simulink model "simulink_model"  (R2015a)
settings: Solver=ode45  StartTime=0.0  StopTime=20  RelTol=1e-3
values from neighbouring files (symbols this model uses):
  g = 9.8    [init_tp.m]    (also in init_tp3.m)
  J = 0.02    [init_tp.m]    (also in init_tp3.m)
  K = place(A,B,p)    [init_tp.m]    (also in init_tp3.m)
  K2 = place(A2,B2,p2)    [init_tp.m]    (also in init_tp3.m)
  m = 0.6    [init_tp.m]    (also in init_tp3.m)
  sigma = 0.8    [init_tp.m]    (also in init_tp3.m)
  w = ((m*g*g)/((1+sigma)*J))^(1/4)    (= 6.32521402527)    [init_tp.m]    (also in init_tp3.m)
settings Model: Creator=root  LastModifiedBy=root

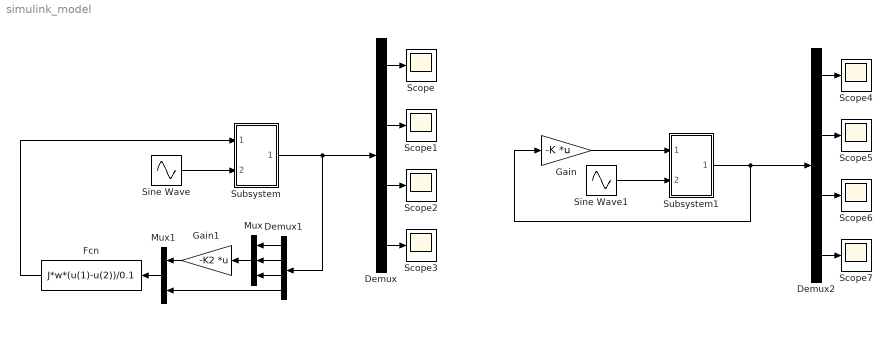
== system simulink_model ==
  Demux : Demux
  Demux1 : Demux
  Demux2 : Demux
  Fcn : Fcn  Expr=J*w*(u(1)-u(2))/0.1
  Gain : Gain  Gain=-K  Multiplication=Matrix(K*u)
  Gain1 : Gain  Gain=-K2  Multiplication=Matrix(K*u)
  Mux : Mux  Inputs=3
  Mux1 : Mux  Inputs=2
  Scope{,1..7} (8 alike) : Scope
      Scope settings: TimeRange=400.0000000000001  YMin=0.05358793969849247  YMax=0.1015879396984925
      Scope2 settings: SaveName=ScopeData2
      Scope3 settings: SaveName=ScopeData3
      Scope4 settings: TimeRange=400.0000000000001  YMin=0.05358793969849247  YMax=0.1015879396984925  SaveName=ScopeData4
      Scope5 settings: SaveName=ScopeData5
      Scope6 settings: SaveName=ScopeData6
      Scope7 settings: SaveName=ScopeData7
  Sine Wave : Sin  Amplitude=0  Frequency=0.1  SampleTime=0
  Sine Wave1 : Sin  Amplitude=0  Frequency=0.1  SampleTime=0
  Subsystem : Subsystem
  Subsystem1 : Subsystem
  wires:
  Demux/1 -> Scope/1
  Demux/2 -> Scope1/1
  Demux/3 -> Scope2/1
  Demux/4 -> Scope3/1
  Subsystem/1(Out1) -> Demux1/1, Demux/1
  Sine Wave/1 -> Subsystem/2(In2)
  Demux1/2 -> Mux/2
  Demux1/3 -> Mux/3
  Demux1/1 -> Mux/1
  Mux/1 -> Gain1/1
  Gain1/1 -> Mux1/1
  Mux1/1 -> Fcn/1
  Demux1/4 -> Mux1/2
  Fcn/1 -> Subsystem/1(In1)
  Demux2/1 -> Scope4/1
  Demux2/2 -> Scope5/1
  Demux2/3 -> Scope6/1
  Demux2/4 -> Scope7/1
  Sine Wave1/1 -> Subsystem1/2(In2)
  Gain/1 -> Subsystem1/1(In1)
  Subsystem1/1(Out1) -> Gain/1, Demux2/1

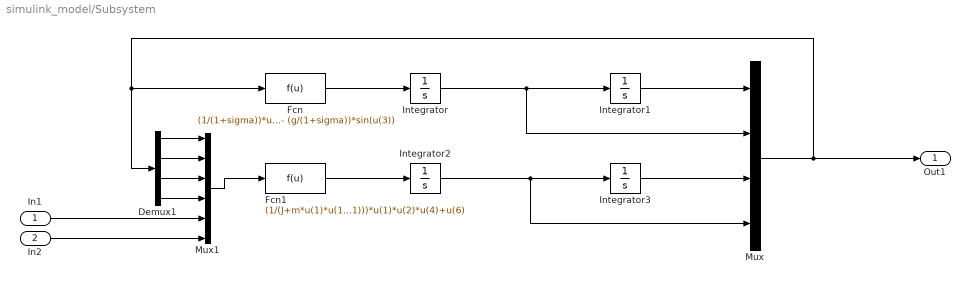
== system simulink_model/Subsystem ==
  In1 : Inport
  In2 : Inport  Port=2
  Demux1 : Demux
  Fcn : Fcn  Expr=(1/(1+sigma))*u(1)*u(4)*u(4) - (g/(1+sigma))*sin(u(3))
  Fcn1 : Fcn  Expr=(1/(J+m*u(1)*u(1)))*u(5) - ((m*g)/(J+m*u(1)*u(1)))*u(1)*cos(u(3)) - ((2*m)/(J+m*u(1)*u(1)))*u(1)*u(2)*u(4)+u(6)
  Integrator : Integrator
  Integrator1 : Integrator  InitialCondition=0.1
  Integrator2 : Integrator
  Integrator3 : Integrator  InitialCondition=0.1
  Mux : Mux
  Mux1 : Mux  Inputs=6
  Out1 : Outport
  wires:
  Demux1/4 -> Mux1/4
  Integrator3/1 -> Mux/3
  Fcn1/1 -> Integrator2/1
  Fcn/1 -> Integrator/1
  Mux/1 -> Out1/1, Demux1/1, Fcn/1
  Demux1/2 -> Mux1/2
  Integrator1/1 -> Mux/1
  Mux1/1 -> Fcn1/1
  Demux1/1 -> Mux1/1
  Integrator2/1 -> Mux/4, Integrator3/1
  Demux1/3 -> Mux1/3
  Integrator/1 -> Mux/2, Integrator1/1
  In1/1 -> Mux1/5
  In2/1 -> Mux1/6

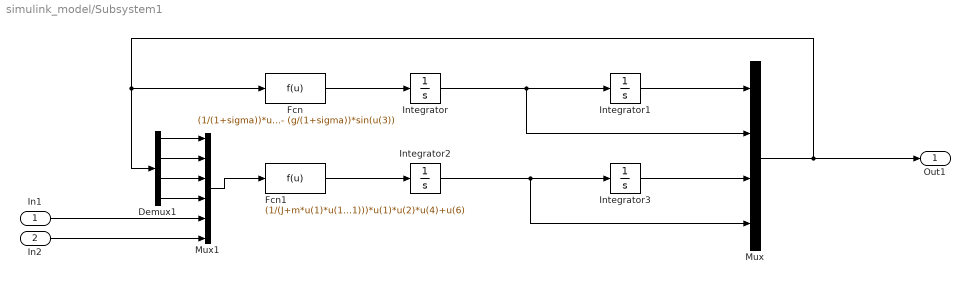
== system simulink_model/Subsystem1 ==
  In1 : Inport
  In2 : Inport  Port=2
  Demux1 : Demux
  Fcn : Fcn  Expr=(1/(1+sigma))*u(1)*u(4)*u(4) - (g/(1+sigma))*sin(u(3))
  Fcn1 : Fcn  Expr=(1/(J+m*u(1)*u(1)))*u(5) - ((m*g)/(J+m*u(1)*u(1)))*u(1)*cos(u(3)) - ((2*m)/(J+m*u(1)*u(1)))*u(1)*u(2)*u(4)+u(6)
  Integrator : Integrator
  Integrator1 : Integrator  InitialCondition=0.1
  Integrator2 : Integrator
  Integrator3 : Integrator  InitialCondition=0.1
  Mux : Mux
  Mux1 : Mux  Inputs=6
  Out1 : Outport
  wires:
  Demux1/4 -> Mux1/4
  Integrator3/1 -> Mux/3
  Fcn1/1 -> Integrator2/1
  Fcn/1 -> Integrator/1
  Mux/1 -> Out1/1, Demux1/1, Fcn/1
  Demux1/2 -> Mux1/2
  Integrator1/1 -> Mux/1
  Mux1/1 -> Fcn1/1
  Demux1/1 -> Mux1/1
  Integrator2/1 -> Mux/4, Integrator3/1
  Demux1/3 -> Mux1/3
  Integrator/1 -> Mux/2, Integrator1/1
  In1/1 -> Mux1/5
  In2/1 -> Mux1/6
